simulink model "Gravity_Compensation_2R_NP"  (R2023a)
settings: Solver=VariableStepAuto  StartTime=0.0  StopTime=10.0  RelTol=1e-3
undefined symbols (not defined in the file): X, Y, Z
libraries: nesl_utility x33, sm_lib x25
settings Model: Creator=manu  LastModifiedBy=deluc
settings DebuggingCC: UnconnectedInputMsg=warning  UnconnectedOutputMsg=warning  UnconnectedLineMsg=warning
settings ModelReferenceCC: EnableRefExpFcnMdlSchedulingChecks=on
settings RTWCC: DLArmComputeVersion=19.05

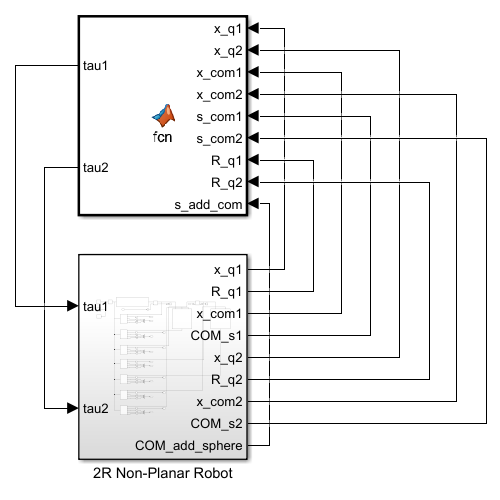
[thumbnail: Simulink's stored preview of the top-level diagram]
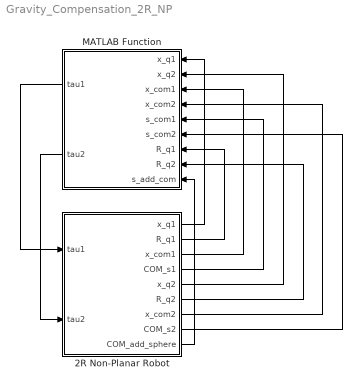
== system Gravity_Compensation_2R_NP ==
  2R Non-Planar Robot : Subsystem
  MATLAB Function : MATLAB Function  TreatAsAtomicUnit=on
  wires:
  MATLAB Function/1(tau1) -> 2R Non-Planar Robot/1(tau1)
  2R Non-Planar Robot/1(x_q1) -> MATLAB Function/1(x_q1)
  2R Non-Planar Robot/2(R_q1) -> MATLAB Function/7(R_q1)
  2R Non-Planar Robot/3(x_com1) -> MATLAB Function/3(x_com1)
  2R Non-Planar Robot/4(COM_s1) -> MATLAB Function/5(s_com1)
  2R Non-Planar Robot/5(x_q2) -> MATLAB Function/2(x_q2)
  2R Non-Planar Robot/7(x_com2) -> MATLAB Function/4(x_com2)
  2R Non-Planar Robot/8(COM_s2) -> MATLAB Function/6(s_com2)
  2R Non-Planar Robot/6(R_q2) -> MATLAB Function/8(R_q2)
  MATLAB Function/2(tau2) -> 2R Non-Planar Robot/2(tau2)
  2R Non-Planar Robot/9(COM_add_sphere) -> MATLAB Function/9(s_add_com)

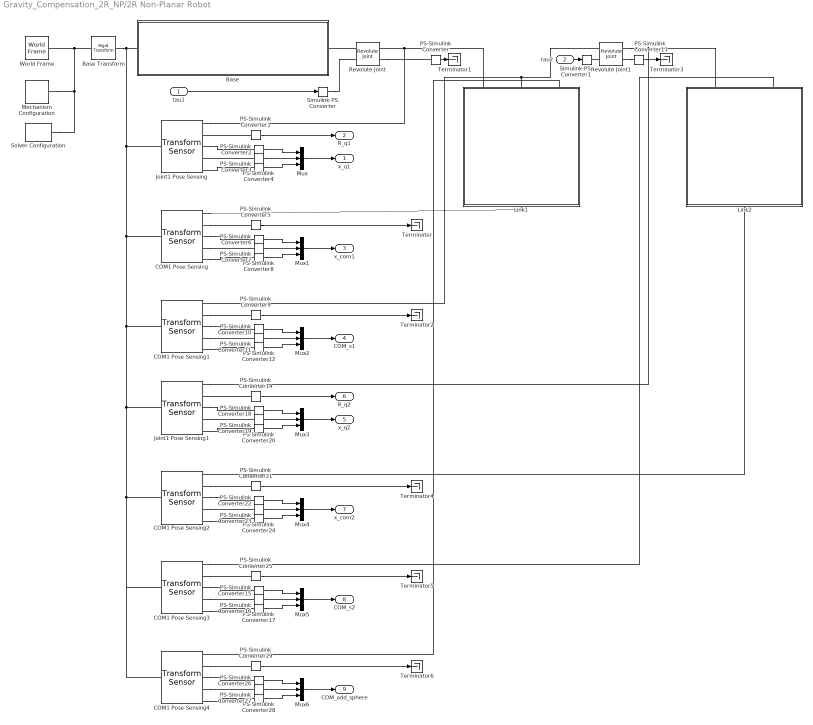
== system Gravity_Compensation_2R_NP/2R Non-Planar Robot ==
  tau1 : Inport
  tau2 : Inport  Port=2
  Base : Subsystem
  Base Transform : sm_lib/Frames and Transforms/Rigid Transform  TranslationMethod=None  TranslationStandardOffset=0  TranslationStandardOffsetUnits=m  TranslationStandardAxis=+Z  TranslationCartesianOffset=[0 0 0]  TranslationCartesianOffsetUnits=m  TranslationROffset=0  TranslationROffsetUnits=m  TranslationZOffset=0  TranslationZOffsetUnits=m  TranslationThetaOffset=0  TranslationThetaOffsetUnits=deg  RotationMethod=AlignedAxes  RotationAngleUnits=deg  RotationStandardAxis=+Z  RotationAngle=0.0  RotationArbitraryAxis=[0 0 1]  FollAlignAxisA=+Z  BaseAlignAxisA=-Y  FollAlignAxisB=+X  BaseAlignAxisB=+X  RotationSequenceAxes=FollowerAxes  RotationSequence=XYX  RotationSequenceAngles=[0 0 0]  RotationSequenceAnglesUnits=deg  RotationMatrix=[1 0 0; 0 1 0; 0 0 1]  Quaternion=[1 0 0 0]
  COM1 Pose Sensing{,1..4} (5 alike) : sm_lib/Frames and Transforms/Transform Sensor  MeasurementFrame=Base  RotationSequence=XYX  SenseAngle=off  SenseAxis=off  SenseQ=off  SenseR=on  SenseRotationSequence=off  SenseOmegaX=off  SenseOmegaY=off  SenseOmegaZ=off  SenseQDot=off  SenseRDot=off  SenseRotationSequenceDot=off  SenseAlphaX=off  SenseAlphaY=off  SenseAlphaZ=off  SenseQDDot=off  SenseRDDot=off  SenseX=on  SenseY=on  SenseZ=on  SenseRad=off  SenseAzim=off  SenseDist=off  SenseInc=off  SenseXDot=off  SenseYDot=off  SenseZDot=off  SenseRadDot=off  SenseAzimDot=off  SenseDistDot=off  SenseIncDot=off  SenseXDDot=off  SenseYDDot=off  SenseZDDot=off  SenseRadDDot=off  SenseAzimDDot=off  SenseDistDDot=off  SenseIncDDot=off
  Joint1 Pose Sensing : sm_lib/Frames and Transforms/Transform Sensor  MeasurementFrame=Base  RotationSequence=XYX  SenseAngle=off  SenseAxis=off  SenseQ=off  SenseR=on  SenseRotationSequence=off  SenseOmegaX=off  SenseOmegaY=off  SenseOmegaZ=off  SenseQDot=off  SenseRDot=off  SenseRotationSequenceDot=off  SenseAlphaX=off  SenseAlphaY=off  SenseAlphaZ=off  SenseQDDot=off  SenseRDDot=off  SenseX=on  SenseY=on  SenseZ=on  SenseRad=off  SenseAzim=off  SenseDist=off  SenseInc=off  SenseXDot=off  SenseYDot=off  SenseZDot=off  SenseRadDot=off  SenseAzimDot=off  SenseDistDot=off  SenseIncDot=off  SenseXDDot=off  SenseYDDot=off  SenseZDDot=off  SenseRadDDot=off  SenseAzimDDot=off  SenseDistDDot=off  SenseIncDDot=off
  Joint1 Pose Sensing1 : sm_lib/Frames and Transforms/Transform Sensor  MeasurementFrame=Base  RotationSequence=XYX  SenseAngle=off  SenseAxis=off  SenseQ=off  SenseR=on  SenseRotationSequence=off  SenseOmegaX=off  SenseOmegaY=off  SenseOmegaZ=off  SenseQDot=off  SenseRDot=off  SenseRotationSequenceDot=off  SenseAlphaX=off  SenseAlphaY=off  SenseAlphaZ=off  SenseQDDot=off  SenseRDDot=off  SenseX=on  SenseY=on  SenseZ=on  SenseRad=off  SenseAzim=off  SenseDist=off  SenseInc=off  SenseXDot=off  SenseYDot=off  SenseZDot=off  SenseRadDot=off  SenseAzimDot=off  SenseDistDot=off  SenseIncDot=off  SenseXDDot=off  SenseYDDot=off  SenseZDDot=off  SenseRadDDot=off  SenseAzimDDot=off  SenseDistDDot=off  SenseIncDDot=off
  Link1 : Subsystem
  Link2 : Subsystem
  Mechanism Configuration : sm_lib/Utilities/Mechanism Configuration  UniformGravity=Constant  GravityVector=[0 0 -9.81]  GravityVectorUnits=m/s^2  LinearizationDelta=0.001  JointModeTransitionNonlinearIterations=2
  Mux{,1..6} (7 alike) : Mux  Inputs=3
  PS-Simulink Converter{,1..29} (30 alike) : nesl_utility/PS-Simulink Converter  PhysicalDomain=network_engine_domain  SubClassName=ps_output  LeftPortType=input  RightPortType=output  PseudoPeriodic=off  Frequencies=[]  VectorFormat=1-D array  Unit=inherit  AffineConversion=off
  Revolute Joint : sm_lib/Joints/Revolute Joint  JointMode=Normal  SenseConstraintForce=off  SenseConstraintForceX=off  SenseConstraintForceY=off  SenseConstraintForceZ=off  SenseConstraintTorque=off  SenseConstraintTorqueX=off  SenseConstraintTorqueY=off  SenseConstraintTorqueZ=off  SenseTotalForce=off  SenseTotalForceX=off  SenseTotalForceY=off  SenseTotalForceZ=off  SenseTotalTorque=off  SenseTotalTorqueX=off  SenseTotalTorqueY=off  SenseTotalTorqueZ=off  CompositeWrenchDir=FollowerOnBase  CompositeWrenchFrame=BaseFrame  EquilibriumPosition=0  EquilibriumPositionUnits=rad  SpringStiffness=0  SpringStiffnessUnits=N*m/rad  DampingCoefficient=0.002  DampingCoefficientUnits=N*m/(rad/s)  TorqueActuationMode=InputTorque  MotionActuationMode=ComputedMotion  SensePosition=on  SenseVelocity=off  SenseAcceleration=off  SenseTorqueForce=off  SenseLowerLimitTorqueForce=off  SenseUpperLimitTorqueForce=off  LowerLimitSpecify=off  LowerLimitBound=-90  LowerLimitBoundUnits=deg  LowerLimitStiffness=1e4  LowerLimitStiffnessUnits=N*m/deg  LowerLimitDamping=10  LowerLimitDampingUnits=N*m/(deg/s)  LowerLimitTransitionRegionWidth=0.1  LowerLimitTransitionRegionWidthUnits=deg  UpperLimitSpecify=off  UpperLimitBound=90  UpperLimitBoundUnits=deg  UpperLimitStiffness=1e4  UpperLimitStiffnessUnits=N*m/deg  UpperLimitDamping=10  UpperLimitDampingUnits=N*m/(deg/s)  UpperLimitTransitionRegionWidth=0.1  UpperLimitTransitionRegionWidthUnits=deg  PositionTargetSpecify=on  PositionTargetPriority=High  PositionTargetValue=30  PositionTargetValueUnits=deg  VelocityTargetSpecify=off  VelocityTargetPriority=High  VelocityTargetValue=0  VelocityTargetValueUnits=deg/s
  Revolute Joint1 : sm_lib/Joints/Revolute Joint  JointMode=Normal  SenseConstraintForce=off  SenseConstraintForceX=off  SenseConstraintForceY=off  SenseConstraintForceZ=off  SenseConstraintTorque=off  SenseConstraintTorqueX=off  SenseConstraintTorqueY=off  SenseConstraintTorqueZ=off  SenseTotalForce=off  SenseTotalForceX=off  SenseTotalForceY=off  SenseTotalForceZ=off  SenseTotalTorque=off  SenseTotalTorqueX=off  SenseTotalTorqueY=off  SenseTotalTorqueZ=off  CompositeWrenchDir=FollowerOnBase  CompositeWrenchFrame=BaseFrame  EquilibriumPosition=0  EquilibriumPositionUnits=rad  SpringStiffness=0  SpringStiffnessUnits=N*m/rad  DampingCoefficient=0.002  DampingCoefficientUnits=N*m/(rad/s)  TorqueActuationMode=InputTorque  MotionActuationMode=ComputedMotion  SensePosition=on  SenseVelocity=off  SenseAcceleration=off  SenseTorqueForce=off  SenseLowerLimitTorqueForce=off  SenseUpperLimitTorqueForce=off  LowerLimitSpecify=off  LowerLimitBound=-90  LowerLimitBoundUnits=deg  LowerLimitStiffness=1e4  LowerLimitStiffnessUnits=N*m/deg  LowerLimitDamping=10  LowerLimitDampingUnits=N*m/(deg/s)  LowerLimitTransitionRegionWidth=0.1  LowerLimitTransitionRegionWidthUnits=deg  UpperLimitSpecify=off  UpperLimitBound=90  UpperLimitBoundUnits=deg  UpperLimitStiffness=1e4  UpperLimitStiffnessUnits=N*m/deg  UpperLimitDamping=10  UpperLimitDampingUnits=N*m/(deg/s)  UpperLimitTransitionRegionWidth=0.1  UpperLimitTransitionRegionWidthUnits=deg  PositionTargetSpecify=on  PositionTargetPriority=High  PositionTargetValue=-30  PositionTargetValueUnits=deg  VelocityTargetSpecify=off  VelocityTargetPriority=High  VelocityTargetValue=0  VelocityTargetValueUnits=deg/s
  Simulink-PS Converter : nesl_utility/Simulink-PS Converter  PhysicalDomain=network_engine_domain  SubClassName=ps_input  LeftPortType=input  RightPortType=output  PseudoPeriodic=off  Frequencies=[]  NoiseDistribution=none  NoiseParameters=[]  Unit=1  AffineConversion=off  FilteringAndDerivatives=provide  SimscapeFilterOrder=1  InputFilterTimeConstant=0.001  UdotUserProvided=0
  Simulink-PS Converter1 : nesl_utility/Simulink-PS Converter  PhysicalDomain=network_engine_domain  SubClassName=ps_input  LeftPortType=input  RightPortType=output  PseudoPeriodic=off  Frequencies=[]  NoiseDistribution=none  NoiseParameters=[]  Unit=1  AffineConversion=off  FilteringAndDerivatives=provide  SimscapeFilterOrder=1  InputFilterTimeConstant=0.001  UdotUserProvided=0
  Solver Configuration : nesl_utility/Solver Configuration  PhysicalDomain=network_engine_domain  SubClassName=solver  LeftPortType=input  RightPortType=generic  Tones=[]  Harmonics=[]  SimulateNoise=off  Profile=off  UseLocalSampling=off  EnableSwitchedLinearOptims=on  FrequencyDomain=off  UseCCode=off  RelTol=0.001  AbsTol=1e-06  MinStep=1e-09  ToWorkspace=off  RevertToSquareIcSolve=off  NumHomotopyIterations=100  PhasorMode=off  PhasorModeNumHarmonics=1  ConsistencySolver=NEWTON_FTOL  IndexReductionMethod=DerivativeReplacement  DoDC=off  ResidualTolerance=1e-09  ConsistencyTolSource=GLOBAL  ConsistencyAbsTol=0.001  ConsistencyRelTol=0.001  ConsistencyTolFactor=0.001  UseLocalSolver=off  LocalSolverChoice=NE_BACKWARD_EULER_ADVANCER  ResolveIndetEquations=on  FunctionEvalNumThread=1  LocalSolverSampleTime=0.001  DoFixedCost=off  MaxNonlinIter=3  MaxModeIter=2  ComputeImpulses=off  ImpulseIterations=2  LinearAlgebra=Sparse  LinearAlgebraNumThread=0  EquationFormulation=NE_TIME_EF  DelaysMemoryBudget=1024  AutomaticFiltering=on  FilteringTimeConstant=0.001  PartitionStorageMethod=AS_NEEDED  PartitionMemoryBudget=1024  PartitionMethod=ROBUST
  Terminator{,1..6} (7 alike) : Terminator
  World Frame : sm_lib/Frames and Transforms/World Frame
  x_q1 : Outport
  R_q1 : Outport  Port=2
  x_com1 : Outport  Port=3
  COM_s1 : Outport  Port=4
  x_q2 : Outport  Port=5
  R_q2 : Outport  Port=6
  x_com2 : Outport  Port=7
  COM_s2 : Outport  Port=8
  COM_add_sphere : Outport  Port=9
  wires:
  PS-Simulink Converter5/1 -> Terminator/1
  Mux1/1 -> x_com1/1
  PS-Simulink Converter8/1 -> Mux1/2
  PS-Simulink Converter7/1 -> Mux1/3
  PS-Simulink Converter1/1 -> R_q1/1
  PS-Simulink Converter6/1 -> Mux1/1
  PS-Simulink Converter/1 -> Terminator1/1
  PS-Simulink Converter3/1 -> Mux/3
  Mux/1 -> x_q1/1
  tau1/1 -> Simulink-PS Converter/1
  PS-Simulink Converter2/1 -> Mux/1
  PS-Simulink Converter4/1 -> Mux/2
  PS-Simulink Converter11/1 -> Mux2/3
  PS-Simulink Converter12/1 -> Mux2/2
  PS-Simulink Converter10/1 -> Mux2/1
  Mux2/1 -> COM_s1/1
  PS-Simulink Converter9/1 -> Terminator2/1
  tau2/1 -> Simulink-PS Converter1/1
  PS-Simulink Converter13/1 -> Terminator3/1
  PS-Simulink Converter25/1 -> Terminator5/1
  PS-Simulink Converter15/1 -> Mux5/1
  PS-Simulink Converter17/1 -> Mux5/2
  PS-Simulink Converter16/1 -> Mux5/3
  Mux3/1 -> x_q2/1
  PS-Simulink Converter18/1 -> Mux3/1
  Mux4/1 -> x_com2/1
  PS-Simulink Converter20/1 -> Mux3/2
  Mux5/1 -> COM_s2/1
  PS-Simulink Converter21/1 -> Terminator4/1
  PS-Simulink Converter23/1 -> Mux4/3
  PS-Simulink Converter14/1 -> R_q2/1
  PS-Simulink Converter24/1 -> Mux4/2
  PS-Simulink Converter19/1 -> Mux3/3
  PS-Simulink Converter22/1 -> Mux4/1
  Mux6/1 -> COM_add_sphere/1
  PS-Simulink Converter28/1 -> Mux6/2
  PS-Simulink Converter26/1 -> Mux6/1
  PS-Simulink Converter29/1 -> Terminator6/1
  PS-Simulink Converter27/1 -> Mux6/3
  connections:
  Revolute Joint/RConn2 -- PS-Simulink Converter/LConn1
  Revolute Joint/LConn1 -- Base/RConn1
  COM1 Pose Sensing/RConn4 -- PS-Simulink Converter8/LConn1
  COM1 Pose Sensing/RConn3 -- PS-Simulink Converter6/LConn1
  COM1 Pose Sensing/RConn2 -- PS-Simulink Converter5/LConn1
  COM1 Pose Sensing2/LConn1 -- COM1 Pose Sensing4/LConn1 -- COM1 Pose Sensing3/LConn1 -- Joint1 Pose Sensing1/LConn1 -- COM1 Pose Sensing1/LConn1 -- Base Transform/RConn1 -- Base/LConn1 -- Joint1 Pose Sensing/LConn1 -- COM1 Pose Sensing/LConn1
  PS-Simulink Converter1/LConn1 -- Joint1 Pose Sensing/RConn2
  PS-Simulink Converter3/LConn1 -- Joint1 Pose Sensing/RConn5
  Link1/LConn1 -- Joint1 Pose Sensing/RConn1 -- Revolute Joint/RConn1
  Mechanism Configuration/RConn1 -- Solver Configuration/RConn1 -- Base Transform/LConn1 -- World Frame/RConn1
  PS-Simulink Converter4/LConn1 -- Joint1 Pose Sensing/RConn4
  COM1 Pose Sensing/RConn5 -- PS-Simulink Converter7/LConn1
  Simulink-PS Converter/RConn1 -- Revolute Joint/LConn2
  Joint1 Pose Sensing/RConn3 -- PS-Simulink Converter2/LConn1
  COM1 Pose Sensing1/RConn5 -- PS-Simulink Converter11/LConn1
  COM1 Pose Sensing1/RConn4 -- PS-Simulink Converter12/LConn1
  COM1 Pose Sensing1/RConn3 -- PS-Simulink Converter10/LConn1
  COM1 Pose Sensing1/RConn2 -- PS-Simulink Converter9/LConn1
  COM1 Pose Sensing/RConn1 -- Link1/RConn1
  Link1/LConn2 -- Revolute Joint1/LConn1 -- COM1 Pose Sensing1/RConn1
  Revolute Joint1/RConn1 -- Joint1 Pose Sensing1/RConn1 -- Link2/LConn1
  Revolute Joint1/LConn2 -- Simulink-PS Converter1/RConn1
  Revolute Joint1/RConn2 -- PS-Simulink Converter13/LConn1
  COM1 Pose Sensing3/RConn5 -- PS-Simulink Converter16/LConn1
  PS-Simulink Converter19/LConn1 -- Joint1 Pose Sensing1/RConn5
  COM1 Pose Sensing3/RConn2 -- PS-Simulink Converter25/LConn1
  COM1 Pose Sensing3/RConn3 -- PS-Simulink Converter15/LConn1
  PS-Simulink Converter20/LConn1 -- Joint1 Pose Sensing1/RConn4
  Joint1 Pose Sensing1/RConn3 -- PS-Simulink Converter18/LConn1
  PS-Simulink Converter14/LConn1 -- Joint1 Pose Sensing1/RConn2
  COM1 Pose Sensing2/RConn2 -- PS-Simulink Converter21/LConn1
  COM1 Pose Sensing2/RConn3 -- PS-Simulink Converter22/LConn1
  COM1 Pose Sensing3/RConn4 -- PS-Simulink Converter17/LConn1
  COM1 Pose Sensing2/RConn5 -- PS-Simulink Converter23/LConn1
  COM1 Pose Sensing2/RConn4 -- PS-Simulink Converter24/LConn1
  Link2/RConn1 -- COM1 Pose Sensing2/RConn1
  COM1 Pose Sensing3/RConn1 -- Link2/LConn2
  COM1 Pose Sensing4/RConn5 -- PS-Simulink Converter27/LConn1
  COM1 Pose Sensing4/RConn4 -- PS-Simulink Converter28/LConn1
  COM1 Pose Sensing4/RConn2 -- PS-Simulink Converter29/LConn1
  COM1 Pose Sensing4/RConn3 -- PS-Simulink Converter26/LConn1
  Link1/LConn3 -- COM1 Pose Sensing4/RConn1

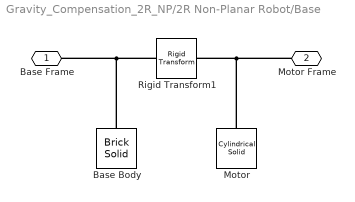
== system Gravity_Compensation_2R_NP/2R Non-Planar Robot/Base ==
  Base Body : sm_lib/Body Elements/Brick Solid  GraphicAmbientColor=[0.15 0.15 0.15 1.0]  BasedOnType=Density  BrickDimensions=[30 30 10]  BrickDimensionsUnits=cm  CenterOfMass=[0 0 0]  CenterOfMassUnits=m  GraphicDiffuseColor=[0.5 0.5 0.5]  Density=1000  DensityUnits=kg/m^3  DoExposeReferenceFrame=on  GraphicEmissiveColor=[0.0 0.0 0.0 1.0]  ExportEntireGeometry=off  SerializedFrames=<Frames/>  MarkerShape=Sphere  MarkerSize=10  GraphicType=FromGeometry  InertiaType=CalculateFromGeometry  Mass=1  MassUnits=kg  MomentsOfInertia=[1 1 1]  MomentsOfInertiaUnits=kg*m^2  GraphicOpacity=1.0  ProductsOfInertia=[0 0 0]  ProductsOfInertiaUnits=kg*m^2  GraphicShininess=75  GraphicSpecularColor=[0.5 0.5 0.5 1.0]  GraphicVisPropType=SimpleVisualProperties
  Motor : sm_lib/Body Elements/Cylindrical Solid  GraphicAmbientColor=[0.15 0.15 0.15 1.0]  BasedOnType=Density  CenterOfMass=[0 0 0]  CenterOfMassUnits=m  GraphicDiffuseColor=[0.0 0.0 0.0]  CylinderLength=10  CylinderLengthUnits=cm  CylinderRadius=5  CylinderRadiusUnits=cm  Density=1000  DensityUnits=kg/m^3  DoExposeReferenceFrame=on  GraphicEmissiveColor=[0.0 0.0 0.0 1.0]  ExportEntireGeometry=off  SerializedFrames=<Frames/>  MarkerShape=Sphere  MarkerSize=10  GraphicType=FromGeometry  InertiaType=CalculateFromGeometry  Mass=1  MassUnits=kg  MomentsOfInertia=[1 1 1]  MomentsOfInertiaUnits=kg*m^2  GraphicOpacity=1.0  ProductsOfInertia=[0 0 0]  ProductsOfInertiaUnits=kg*m^2  GraphicShininess=75  GraphicSpecularColor=[0.5 0.5 0.5 1.0]  GraphicVisPropType=SimpleVisualProperties
  Rigid Transform1 : sm_lib/Frames and Transforms/Rigid Transform  TranslationMethod=StandardAxis  TranslationStandardOffset=10  TranslationStandardOffsetUnits=cm  TranslationStandardAxis=+Z  TranslationCartesianOffset=[0 0 0]  TranslationCartesianOffsetUnits=m  TranslationROffset=0  TranslationROffsetUnits=m  TranslationZOffset=0  TranslationZOffsetUnits=m  TranslationThetaOffset=0  TranslationThetaOffsetUnits=deg  RotationMethod=None  RotationAngleUnits=deg  RotationStandardAxis=+Y  RotationAngle=90  RotationArbitraryAxis=[0 0 1]  FollAlignAxisA=+X  BaseAlignAxisA=+Y  FollAlignAxisB=+Y  BaseAlignAxisB=+Z  RotationSequenceAxes=FollowerAxes  RotationSequence=XYX  RotationSequenceAngles=[0 0 0]  RotationSequenceAnglesUnits=deg  RotationMatrix=[1 0 0; 0 1 0; 0 0 1]  Quaternion=[1 0 0 0]
  Base Frame : PMIOPort  Side=Left
  Motor Frame : PMIOPort  Port=2  Side=Right
  connections:
  Base Body/RConn1 -- Base Frame/RConn1 -- Rigid Transform1/LConn1
  Motor/RConn1 -- Motor Frame/RConn1 -- Rigid Transform1/RConn1

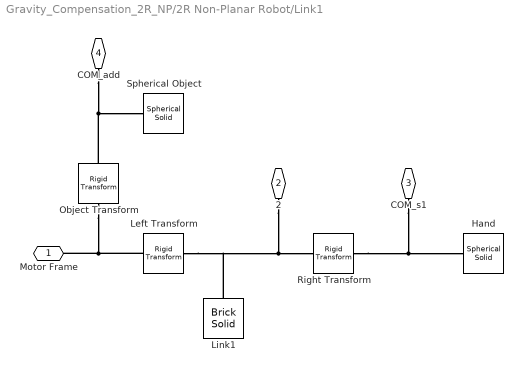
== system Gravity_Compensation_2R_NP/2R Non-Planar Robot/Link1 ==
  Hand : sm_lib/Body Elements/Spherical Solid  GraphicAmbientColor=[0.15 0.15 0.15 1.0]  BasedOnType=Mass  CenterOfMass=[0 0 0]  CenterOfMassUnits=m  GraphicDiffuseColor=[0.2 0.2 1.0]  Density=1000  DensityUnits=kg/m^3  DoExposeReferenceFrame=on  GraphicEmissiveColor=[0.0 0.0 0.0 1.0]  ExportEntireGeometry=off  SerializedExposedGeometries=<ExposedGeometries/>  SerializedFrames=<Frames/>  MarkerShape=Sphere  MarkerSize=10  GraphicType=FromGeometry  InertiaType=CalculateFromGeometry  Mass=0  MassUnits=kg  MomentsOfInertia=[1 1 1]  MomentsOfInertiaUnits=kg*m^2  GraphicOpacity=1.0  ProductsOfInertia=[0 0 0]  ProductsOfInertiaUnits=kg*m^2  GraphicShininess=75  GraphicSpecularColor=[0.5 0.5 0.5 1.0]  SphereRadius=5  SphereRadiusUnits=cm  GraphicVisPropType=SimpleVisualProperties
  Left Transform : sm_lib/Frames and Transforms/Rigid Transform  TranslationMethod=StandardAxis  TranslationStandardOffset=25  TranslationStandardOffsetUnits=cm  TranslationStandardAxis=-X  TranslationCartesianOffset=[0.7 0.5 0]  TranslationCartesianOffsetUnits=m  TranslationROffset=0  TranslationROffsetUnits=m  TranslationZOffset=0  TranslationZOffsetUnits=m  TranslationThetaOffset=0  TranslationThetaOffsetUnits=deg  RotationMethod=None  RotationAngleUnits=deg  RotationStandardAxis=+Z  RotationAngle=38  RotationArbitraryAxis=[0 0 1]  FollAlignAxisA=+X  BaseAlignAxisA=+Y  FollAlignAxisB=+Y  BaseAlignAxisB=+Z  RotationSequenceAxes=FollowerAxes  RotationSequence=XYX  RotationSequenceAngles=[0 0 0]  RotationSequenceAnglesUnits=deg  RotationMatrix=[1 0 0; 0 1 0; 0 0 1]  Quaternion=[1 0 0 0]
  Link1 : sm_lib/Body Elements/Brick Solid  GraphicAmbientColor=[0.15 0.15 0.15 1.0]  BasedOnType=Mass  BrickDimensions=[50 5 5]  BrickDimensionsUnits=cm  CenterOfMass=[0 0 0]  CenterOfMassUnits=m  GraphicDiffuseColor=[1.0 0.0 0.0]  Density=1000  DensityUnits=kg/m^3  DoExposeReferenceFrame=on  GraphicEmissiveColor=[0.0 0.0 0.0 1.0]  ExportEntireGeometry=off  SerializedFrames=<Frames/>  MarkerShape=Sphere  MarkerSize=10  GraphicType=FromGeometry  InertiaType=CalculateFromGeometry  Mass=2  MassUnits=kg  MomentsOfInertia=[1 1 1]  MomentsOfInertiaUnits=kg*m^2  GraphicOpacity=1.0  ProductsOfInertia=[0 0 0]  ProductsOfInertiaUnits=kg*m^2  GraphicShininess=75  GraphicSpecularColor=[0.5 0.5 0.5 1.0]  GraphicVisPropType=SimpleVisualProperties
  Object Transform : sm_lib/Frames and Transforms/Rigid Transform  TranslationMethod=StandardAxis  TranslationStandardOffset=-50*(2/3)  TranslationStandardOffsetUnits=cm  TranslationStandardAxis=+X  TranslationCartesianOffset=[0.7 0.5 0]  TranslationCartesianOffsetUnits=m  TranslationROffset=0  TranslationROffsetUnits=m  TranslationZOffset=0  TranslationZOffsetUnits=m  TranslationThetaOffset=0  TranslationThetaOffsetUnits=deg  RotationMethod=None  RotationAngleUnits=deg  RotationStandardAxis=+Z  RotationAngle=38  RotationArbitraryAxis=[0 0 1]  FollAlignAxisA=+X  BaseAlignAxisA=+Y  FollAlignAxisB=+Y  BaseAlignAxisB=+Z  RotationSequenceAxes=FollowerAxes  RotationSequence=XYX  RotationSequenceAngles=[0 0 0]  RotationSequenceAnglesUnits=deg  RotationMatrix=[1 0 0; 0 1 0; 0 0 1]  Quaternion=[1 0 0 0]
  Right Transform : sm_lib/Frames and Transforms/Rigid Transform  TranslationMethod=StandardAxis  TranslationStandardOffset=25  TranslationStandardOffsetUnits=cm  TranslationStandardAxis=+X  TranslationCartesianOffset=[0 0 0]  TranslationCartesianOffsetUnits=m  TranslationROffset=0  TranslationROffsetUnits=m  TranslationZOffset=0  TranslationZOffsetUnits=m  TranslationThetaOffset=0  TranslationThetaOffsetUnits=deg  RotationMethod=AlignedAxes  RotationAngleUnits=deg  RotationStandardAxis=+Z  RotationAngle=0.0  RotationArbitraryAxis=[0 0 1]  FollAlignAxisA=+Z  BaseAlignAxisA=+X  FollAlignAxisB=+Y  BaseAlignAxisB=+Y  RotationSequenceAxes=FollowerAxes  RotationSequence=XYX  RotationSequenceAngles=[0 0 0]  RotationSequenceAnglesUnits=deg  RotationMatrix=[1 0 0; 0 1 0; 0 0 1]  Quaternion=[1 0 0 0]
  Spherical Object : sm_lib/Body Elements/Spherical Solid  GraphicAmbientColor=[0.15 0.15 0.15 1.0]  BasedOnType=Mass  CenterOfMass=[0 0 0]  CenterOfMassUnits=m  GraphicDiffuseColor=[0.0 0.6 0.0]  Density=1000  DensityUnits=kg/m^3  DoExposeReferenceFrame=on  GraphicEmissiveColor=[0.0 0.0 0.0 1.0]  ExportEntireGeometry=off  SerializedExposedGeometries=<ExposedGeometries/>  SerializedFrames=<Frames/>  MarkerShape=Sphere  MarkerSize=10  GraphicType=FromGeometry  InertiaType=CalculateFromGeometry  Mass=7  MassUnits=kg  MomentsOfInertia=[1 1 1]  MomentsOfInertiaUnits=kg*m^2  GraphicOpacity=1.0  ProductsOfInertia=[0 0 0]  ProductsOfInertiaUnits=kg*m^2  GraphicShininess=75  GraphicSpecularColor=[0.5 0.5 0.5 1.0]  SphereRadius=5  SphereRadiusUnits=cm  GraphicVisPropType=SimpleVisualProperties
  Motor Frame : PMIOPort  Side=Left
  2 : PMIOPort  Port=2  Side=Right
  COM_s1 : PMIOPort  Port=3  Side=Left
  COM_add : PMIOPort  Port=4  Side=Left
  connections:
  2/RConn1 -- Left Transform/LConn1 -- Link1/RConn1 -- Right Transform/LConn1
  Right Transform/RConn1 -- COM_s1/RConn1 -- Hand/RConn1
  Object Transform/RConn1 -- Left Transform/RConn1 -- Motor Frame/RConn1
  Object Transform/LConn1 -- COM_add/RConn1 -- Spherical Object/RConn1

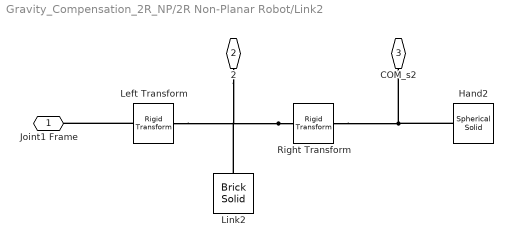
== system Gravity_Compensation_2R_NP/2R Non-Planar Robot/Link2 ==
  Hand2 : sm_lib/Body Elements/Spherical Solid  GraphicAmbientColor=[0.15 0.15 0.15 1.0]  BasedOnType=Mass  CenterOfMass=[0 0 0]  CenterOfMassUnits=m  GraphicDiffuseColor=[0.2 0.2 1.0]  Density=1000  DensityUnits=kg/m^3  DoExposeReferenceFrame=on  GraphicEmissiveColor=[0.0 0.0 0.0 1.0]  ExportEntireGeometry=off  SerializedExposedGeometries=<ExposedGeometries/>  SerializedFrames=<Frames/>  MarkerShape=Sphere  MarkerSize=10  GraphicType=FromGeometry  InertiaType=CalculateFromGeometry  Mass=2  MassUnits=kg  MomentsOfInertia=[1 1 1]  MomentsOfInertiaUnits=kg*m^2  GraphicOpacity=1.0  ProductsOfInertia=[0 0 0]  ProductsOfInertiaUnits=kg*m^2  GraphicShininess=75  GraphicSpecularColor=[0.5 0.5 0.5 1.0]  SphereRadius=5  SphereRadiusUnits=cm  GraphicVisPropType=SimpleVisualProperties
  Left Transform : sm_lib/Frames and Transforms/Rigid Transform  TranslationMethod=StandardAxis  TranslationStandardOffset=15  TranslationStandardOffsetUnits=cm  TranslationStandardAxis=-X  TranslationCartesianOffset=[0.7 0.5 0]  TranslationCartesianOffsetUnits=m  TranslationROffset=0  TranslationROffsetUnits=m  TranslationZOffset=0  TranslationZOffsetUnits=m  TranslationThetaOffset=0  TranslationThetaOffsetUnits=deg  RotationMethod=None  RotationAngleUnits=deg  RotationStandardAxis=+Z  RotationAngle=38  RotationArbitraryAxis=[0 0 1]  FollAlignAxisA=+X  BaseAlignAxisA=+Y  FollAlignAxisB=+Y  BaseAlignAxisB=+Z  RotationSequenceAxes=FollowerAxes  RotationSequence=XYX  RotationSequenceAngles=[0 0 0]  RotationSequenceAnglesUnits=deg  RotationMatrix=[1 0 0; 0 1 0; 0 0 1]  Quaternion=[1 0 0 0]
  Link2 : sm_lib/Body Elements/Brick Solid  GraphicAmbientColor=[0.15 0.15 0.15 1.0]  BasedOnType=Mass  BrickDimensions=[30 5 5]  BrickDimensionsUnits=cm  CenterOfMass=[0 0 0]  CenterOfMassUnits=m  GraphicDiffuseColor=[1.0 0.0 0.0]  Density=1000  DensityUnits=kg/m^3  DoExposeReferenceFrame=on  GraphicEmissiveColor=[0.0 0.0 0.0 1.0]  ExportEntireGeometry=off  SerializedFrames=<Frames/>  MarkerShape=Sphere  MarkerSize=10  GraphicType=FromGeometry  InertiaType=CalculateFromGeometry  Mass=1  MassUnits=kg  MomentsOfInertia=[1 1 1]  MomentsOfInertiaUnits=kg*m^2  GraphicOpacity=1.0  ProductsOfInertia=[0 0 0]  ProductsOfInertiaUnits=kg*m^2  GraphicShininess=75  GraphicSpecularColor=[0.5 0.5 0.5 1.0]  GraphicVisPropType=SimpleVisualProperties
  Right Transform : sm_lib/Frames and Transforms/Rigid Transform  TranslationMethod=StandardAxis  TranslationStandardOffset=15  TranslationStandardOffsetUnits=cm  TranslationStandardAxis=+X  TranslationCartesianOffset=[0 0 0]  TranslationCartesianOffsetUnits=m  TranslationROffset=0  TranslationROffsetUnits=m  TranslationZOffset=0  TranslationZOffsetUnits=m  TranslationThetaOffset=0  TranslationThetaOffsetUnits=deg  RotationMethod=None  RotationAngleUnits=deg  RotationStandardAxis=+Z  RotationAngle=0.0  RotationArbitraryAxis=[0 0 1]  FollAlignAxisA=+X  BaseAlignAxisA=+Y  FollAlignAxisB=+Y  BaseAlignAxisB=+Z  RotationSequenceAxes=FollowerAxes  RotationSequence=XYX  RotationSequenceAngles=[0 0 0]  RotationSequenceAnglesUnits=deg  RotationMatrix=[1 0 0; 0 1 0; 0 0 1]  Quaternion=[1 0 0 0]
  Joint1 Frame : PMIOPort  Side=Left
  2 : PMIOPort  Port=2  Side=Right
  COM_s2 : PMIOPort  Port=3  Side=Left
  connections:
  Right Transform/LConn1 -- 2/RConn1 -- Left Transform/LConn1 -- Link2/RConn1
  Hand2/RConn1 -- Right Transform/RConn1 -- COM_s2/RConn1
  Left Transform/RConn1 -- Joint1 Frame/RConn1

== matlab function Gravity_Compensation_2R_NP/MATLAB Function ==
  data: x_q1 input; x_q2 input; x_com1 input; x_com2 input; s_com1 input; s_com2 input; tau1 output; R_q1 input; R_q2 input; tau2 output; s_add_com input
function [tau1,tau2]= fcn(x_q1,x_q2,x_com1,x_com2,s_com1,s_com2, R_q1, R_q2, s_add_com)
    
    % Define masses of the objects
    m1=2;    % Mass of the links1
    m2=0;    % Mass of the sphere1 (assuming it's negligible)
    m3=1;    % Mass of the links2
    m4=2;    % Mass of the sphere2
    m_add=7; % Mass of the added spherical object
    
    % Define gravitational acceleration along y-axis wrt the base frame
    g=[0; -9.81; 0];
    
    % Calculate gravitational forces on each object
    F1=m1*g;
    F2=m2*g;
    F3=m3*g;
    F4=m4*g;
    F_add=m_add*g;
    
    % Combine forces into a single vector
    F = [F1; F2; F3; F4; F_add];

    % Calculate rotation axes (unit vectors along z-axis) wrt the base frame
    k1=R_q1*[0;0;1]; 
    k2=R_q2*[0;0;1]; 
    
    % Calculate distances from each object's center of mass to the base frame
    r_1_1_l = x_com1-x_q1;  % Distance from link1 to frame1 
    r_1_1_s = s_com1-x_q1;  % Distance from sphere1 to frame1 
    r_2_1_l = x_com2-x_q1;  % Distance from link2 to frame1 
    r_2_1_s = s_com2-x_q1;  % Distance from sphere2 to frame1 
    r_2_2_l = x_com2-x_q2;  % Distance from link2 to frame2
    r_2_2_s = s_com2-x_q2;  % Distance from sphere2 to frame2 
    r_add = s_add_com-x_q1; % Distance from the added sphere to frame1
    
    % Calculate Jacobians for each object
    J_l1 = [cross(k1, r_1_1_l) zeros(3,1)];         % Jacobian for link1
    J_l2 = [cross(k1, r_1_1_s) zeros(3,1)];         % Jacobian for sphere1
    J_l3 = [cross(k1, r_2_1_l) cross(k2, r_2_2_l)]; % Jacobian for link2
    J_l4 = [cross(k1, r_2_1_s) cross(k2, r_2_2_s)]; % Jacoabian for sphere2
    J_add = [cross(k1, r_add) zeros(3,1)];          % Jacobian for the added sphere 
    
    % Combine all Jacobians into a single matrix
    J = [J_l1', J_l2', J_l3', J_l4' , J_add'];
    
    % Calculate torques required for gravity compensation
    tau = -J * F;
    
    % Extract torques for each joint
    tau1 = tau(1,1);
    tau2 = tau(2,1);
end
